simulink model "bloco_Controle"  (R2015a)
settings: Solver=ode45  StartTime=0.0  StopTime=10.0  RelTol=1e-3
settings Model: Creator=YecidMoreno  LastModifiedBy=YecidMoreno

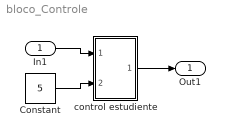
== system bloco_Controle ==
  In1 : Inport
  Constant : Constant  Value=5
  "control estudiente " : Subsystem
  Out1 : Outport
  wires:
  In1/1 -> "control estudiente "/1(In1)
  "control estudiente "/1(Out1) -> Out1/1
  Constant/1 -> "control estudiente "/2(In2)

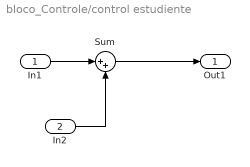
== system bloco_Controle/control estudiente  ==
  In1 : Inport
  In2 : Inport  Port=2
  Sum : Sum  Inputs=|++
  Out1 : Outport
  wires:
  Sum/1 -> Out1/1
  In1/1 -> Sum/1
  In2/1 -> Sum/2
